simulink model "elaborated_design"  (Simulink 7.0)
settings: Solver=ode45  SolverMode=SingleTasking  StartTime=0.0  StopTime=24/3000  RelTol=1e-6
PreLoadFcn:
  | load one_stage.mat
  | load multi_stage.mat
  | generate_fir_lut
undefined symbols (not defined in the file or in its folder): hm, lut_matrix
libraries: simulink x9, dspmlti4 x4, simulink_extras x2, dspsigops x1
(part 1 of 2)
settings Model: Creator=abehbood  LastModifiedBy=abehbood  BufferReuse=off
settings SolverCC: ConsecutiveZCsStepRelTol=128*eps  ZeroCrossControl=DisableAll
settings DataIOCC: LimitDataPoints=off  SaveFormat=StructureWithTime
settings OptimizationCC: OptimizeBlockIOStorage=off  BufferReuse=off  ExpressionFolding=off  LocalBlockOutputs=off
settings DebuggingCC: SaveWithParameterizedLinksMsg=none  SignalResolutionControl=TryResolveAllWithWarning
settings GRTTargetCC: TargetFcnLib=ansi_tfl_tmw.mat

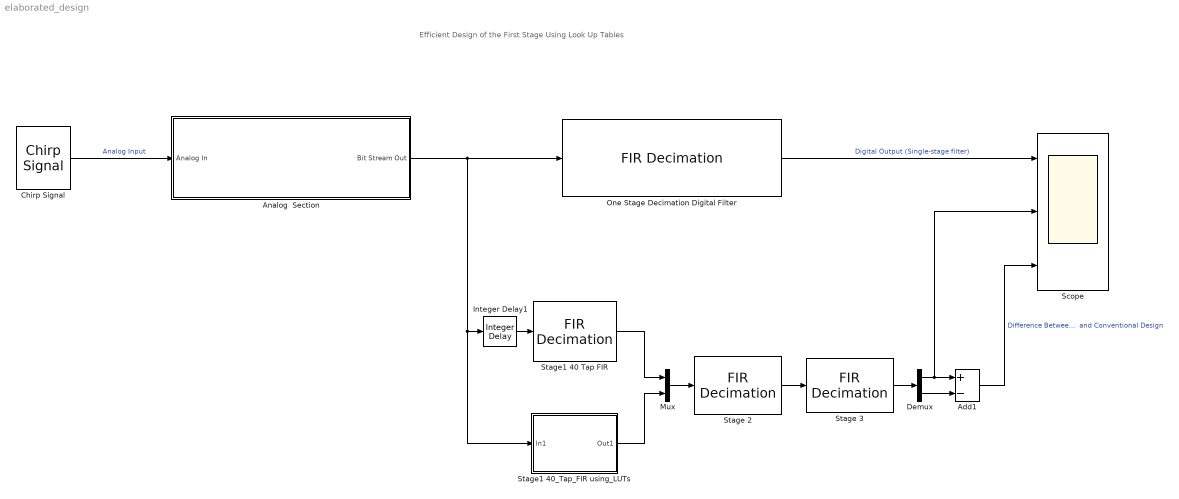
== system elaborated_design ==
  note: Efficient Design of the First Stage
      | Using Look Up Tables
  Add1 : Sum  Inputs=+-  OutDataType=sfix(16)  OutScaling=2^-10
  Analog  Section : Subsystem
  Chirp Signal : simulink/Sources/Chirp Signal  SystemSampleTime=-1  f1=.1  T=6/3000  f2=1000
  Demux : Demux  Outputs=2
  Integer Delay1 : simulink/Discrete/Integer Delay  vinit=0  samptime=-1  NumDelays=1
  Mux : Mux  Inputs=2
  One Stage Decimation Digital Filter : dspmlti4/FIR Decimation  Tag=BlockMethodSubSystem  RequirementInfo={'other' 'AD1877.pdf' '#4' 'true' 'ADI AD1877 Data Sheet' '' } %GIDa_09ac136c_1eca_41b1_bc0b_62c1f7d0b7d0  DialogController=dspdialog.FIRDecimation  DialogControllerArgs=DataTag0  h=[1.55406407911568e-005 -4.02976869344532e-006 -3.62744882919974e-006 -3.32415900794419e-006 -3.10004007346292e-006 -2.94488775900927e-006 -2.84407867825443e-006 -2.79175810569639e-006 -2.77680534274625e-006 -2.79636876946116e-006 -2.84159739559419e-006 -2.91172216432913e-006 -2.99938731666961e-006 -3.10526988821609e-006 -3.22293122491583e-006 -3.35411175577608e-006 -3.49288760841827e-006 -3.64182441067023e-006 -3.79519422790614e-006 -3.95625120366779e-006 -4.11924776887857e-006 -4.28807690784027e-006 -4.45674935295447e-006 -4.62985561457222e-006 -4.800897058436e-006 -4.9753188968358e-006 -5.14579209170125e-006 -5.31896147362731e-006 -5.48613787011061e-006 -5.65584148286576e-006 -5.81687994870294e-006 -5.98156442936665e-006 -6.1319779994032e-006 -6.29670705116336e-006 -6.41916030653874e-006 -6.5873274394144e-006 -6.7177176233061e-006 -6.82652503989139e-006 -6.95495460798152e-006 -7.07534295461106e-006 -7.1850354195168e-006 -7.27502374181979e-006 -7.35666591949478e-006 -7.42908966098812e-006 -7.49731879243244e-006 -7.55554016300166e-006 -7.60384694343128e-006 -7.63736428406282e-006 -7.65751209128601e-006 -7.66271823557677e-006 -7.65541155261304e-006 -7.63501627507501e-006 -7.60282107295533e-006 -7.55771586095076e-006 -7.49955110139743e-006 -7.42707797821989e-006 -7.33956971085392e-006 -7.23653893398005e-006 -7.11727392514411e-006 -6.98238367840012e-006 -6.83104946879514e-006 -6.66483440906746e-006 -6.48225897487408e-006 -6.28578538645417e-006 -6.07254142810829e-006 -5.84668058135014e-006 -5.60212405026277e-006 -5.34827643472346e-006 -5.07102301413336e-006 -4.78659690402004e-006 -4.48580556034723e-006 -4.16155600384522e-006 -3.83401955134294e-006 -3.48874328670483e-006 -3.12800075717904e-006 -2.75159431264472e-006 -2.36710798789534e-006 -1.97052071697094e-006 -1.56289826517329e-006 -1.1415501968765e-006 -7.10846494538715e-007 -2.70732289220279e-007 1.75793679903884e-007 6.30605543525479e-007 1.09226506478532e-006 1.56189731593155e-006 2.03697170915753e-006 2.51723717113145e-006 3.00015723143587e-006 3.48579071809432e-006 3.9725933377886e-006 4.46080384428176e-006 4.9490441253173e-006 5.43679761975195e-006 5.92239585030302e-006 6.40461366377309e-006 6.88208470617973e-006 7.35331974962638e-006 7.81788083672163e-006 8.27366149467831e-006 8.72161880365281e-006 9.15789014754869e-006 9.58466277051695e-006 9.99868488513386e-006 1.03961241773662e-005 1.07845165019174e-005 1.11507237228684e-005 1.1501595755956e-005 1.18347779752421e-005 1.21491508417921e-005 1.24402661260835e-005 1.27113476734474e-005 1.29603423782727e-005 1.31870907689413e-005 1.33876586413025e-005 1.35630197026232e-005 1.37115784405412e-005 1.38343308497875e-005 1.39285220410779e-005 1.39941223446797e-005 1.40289966823036e-005 1.40342134443906e-005 1.40084936488381e-005 1.39526353305602e-005 1.3864821369379e-005 1.37453066068296e-005 1.35925703287186e-005 1.34073463479953e-005 1.3188789625357e-005 1.29377174450497e-005 1.26533131128865e-005 1.23359924862388e-005 1.19851377636711e-005 1.16010858578809e-005 1.11839953027825e-005 1.07344849783013e-005 1.02524591509204e-005 9.74071213530745e-006 9.19501972815777e-006 8.62303106439748e-006 8.0182133965873e-006 7.38519650181956e-006 6.72464037253548e-006 6.03717286198122e-006 5.32193639834688e-006 4.58308951056204e-006 3.82060966862603e-006 3.03594631004846e-006 2.22877471347222e-006 1.40249577164911e-006 5.57771396078279e-007 -3.03081212010611e-007 -1.18011136255105e-006 -2.0703284116168e-006 -2.97257001796215e-006 -3.8836096780257e-006 -4.80290798314314e-006 -5.72785477296596e-006 -6.65770229898759e-006 -7.58923677050474e-006 -8.52121235074221e-006 -9.45049303838782e-006 -1.03761550722017e-005 -1.12952557815384e-005 -1.22066400703126e-005 -1.31069929510391e-005 -1.39948646063552e-005 -1.48669844016962e-005 -1.5722291797911e-005 -1.6557361960285e-005 -1.73721743499725e-005 -1.81614198379814e-005 -1.89271227804299e-005 -1.96621709077627e-005 -2.03681220570147e-005 -2.10414746689456e-005 -2.16795973059757e-005 ...(+43466 chars)]  D=64  filtStruct=Direct form  framing=Maintain input frame size  outputBufInitCond=0  roundingMode=Floor  overflowMode=off  FilterSource=Filter object  FilterObject=h
  Scope : Scope  NumInputPorts=3
      settings: TimeRange=0.008  YMin=-2~-2~-0.2  YMax=2~2~0.2
  Stage 2 : dspmlti4/FIR Decimation  Tag=BlockMethodSubSystem  DialogController=dspdialog.FIRDecimation  DialogControllerArgs=DataTag1  h=[0.006011962890625 -0.0025787353515625 -0.0494384765625 0.0092315673828125 0.293411254882813 0.486648559570313 0.293411254882813 0.0092315673828125 -0.0494384765625 -0.0025787353515625 0.006011962890625]  D=2  filtStruct=Direct form  framing=Maintain input frame size  outputBufInitCond=0  firstCoeffMode=Binary point scaling  firstCoeffWordLength=16  firstCoeffFracLength=16  outputMode=Binary point scaling  outputWordLength=16  outputFracLength=15  accumMode=Binary point scaling  accumWordLength=33  accumFracLength=31  prodOutputMode=Binary point scaling  prodOutputWordLength=31  prodOutputFracLength=31  roundingMode=Nearest  overflowMode=off  FilterSource=Filter object  FilterObject=hm.stage(2)
  Stage 3 : dspmlti4/FIR Decimation  Tag=BlockMethodSubSystem  DialogController=dspdialog.FIRDecimation  DialogControllerArgs=DataTag2  h=[-2.288818359375e-005 -7.62939453125e-006 1.52587890625e-005 4.57763671875e-005 8.392333984375e-005 8.392333984375e-005 3.814697265625e-005 -5.340576171875e-005 -0.0001373291015625 -0.0001678466796875 -9.918212890625e-005 5.340576171875e-005 0.0002288818359375 0.00031280517578125 0.00022125244140625 -3.0517578125e-005 -0.000335693359375 -0.000518798828125 -0.00043487548828125 -6.103515625e-005 0.00045013427734375 0.0008087158203125 0.00077056884765625 0.00025177001953125 -0.00054168701171875 -0.0011749267578125 -0.001251220703125 -0.000579833984375 0.00057220458984375 0.001617431640625 0.0019073486328125 0.0011138916015625 -0.00048828125 -0.002105712890625 -0.00276947021484375 -0.00191497802734375 0.0002288818359375 0.0026092529296875 0.0038604736328125 0.0030517578125 0.00031280517578125 -0.0030670166015625 -0.00519561767578125 -0.0046234130859375 -0.0012359619140625 0.00341033935546875 0.00679779052734375 0.006744384765625 0.00272369384765625 -0.00353240966796875 -0.008697509765625 -0.00959014892578125 -0.00499725341796875 0.00327301025390625 0.0109710693359375 0.0134963989257813 0.0084991455078125 -0.00238037109375 -0.0137939453125 -0.0191268920898438 -0.01409912109375 0.0003662109375 0.0176849365234375 0.028228759765625 0.0241317749023438 0.0041046142578125 -0.0243759155273438 -0.0468978881835938 -0.0477294921875 -0.0169906616210938 0.0438156127929688 0.120735168457031 0.191574096679688 0.233955383300781 0.233955383300781 0.191574096679688 0.120735168457031 0.0438156127929688 -0.0169906616210938 -0.0477294921875 -0.0468978881835938 -0.0243759155273438 0.0041046142578125 0.0241317749023438 0.028228759765625 0.0176849365234375 0.0003662109375 -0.01409912109375 -0.0191268920898438 -0.0137939453125 -0.00238037109375 0.0084991455078125 0.0134963989257813 0.0109710693359375 0.00327301025390625 -0.00499725341796875 -0.00959014892578125 -0.008697509765625 -0.00353240966796875 0.00272369384765625 0.006744384765625 0.00679779052734375 0.00341033935546875 -0.0012359619140625 -0.0046234130859375 -0.00519561767578125 -0.0030670166015625 0.00031280517578125 0.0030517578125 0.0038604736328125 0.0026092529296875 0.0002288818359375 -0.00191497802734375 -0.00276947021484375 -0.002105712890625 -0.00048828125 0.0011138916015625 0.0019073486328125 0.001617431640625 0.00057220458984375 -0.000579833984375 -0.001251220703125 -0.0011749267578125 -0.00054168701171875 0.00025177001953125 0.00077056884765625 0.0008087158203125 0.00045013427734375 -6.103515625e-005 -0.00043487548828125 -0.000518798828125 -0.000335693359375 -3.0517578125e-005 0.00022125244140625 0.00031280517578125 0.0002288818359375 5.340576171875e-005 -9.918212890625e-005 -0.0001678466796875 -0.0001373291015625 -5.340576171875e-005 3.814697265625e-005 8.392333984375e-005 8.392333984375e-005 4.57763671875e-005 1.52587890625e-005 -7.62939453125e-006 -2.288818359375e-005]  D=4  filtStruct=Direct form  framing=Maintain input frame size  outputBufInitCond=0  firstCoeffMode=Binary point scaling  firstCoeffWordLength=16  firstCoeffFracLength=17  outputMode=Binary point scaling  outputWordLength=16  outputFracLength=15  accumMode=Binary point scaling  accumWordLength=34  accumFracLength=32  prodOutputMode=Binary point scaling  prodOutputWordLength=31  prodOutputFracLength=32  roundingMode=Nearest  overflowMode=off  FilterSource=Filter object  FilterObject=hm.stage(3)
  Stage1 40 Tap FIR : dspmlti4/FIR Decimation  Tag=BlockMethodSubSystem  DialogController=dspdialog.FIRDecimation  DialogControllerArgs=DataTag3  h=[-9.5367431640625e-005 -0.00032806396484375 -0.00081634521484375 -0.00164794921875 -0.00287246704101563 -0.004425048828125 -0.00608062744140625 -0.007415771484375 -0.0078125 -0.0065155029296875 -0.00275421142578125 0.00410842895507813 0.0143890380859375 0.0279426574707031 0.0440788269042969 0.0615692138671875 0.0787696838378906 0.0938453674316406 0.105056762695313 0.111034393310547 0.111034393310547 0.105056762695313 0.0938453674316406 0.0787696838378906 0.0615692138671875 0.0440788269042969 0.0279426574707031 0.0143890380859375 0.00410842895507813 -0.00275421142578125 -0.0065155029296875 -0.0078125 -0.007415771484375 -0.00608062744140625 -0.004425048828125 -0.00287246704101563 -0.00164794921875 -0.00081634521484375 -0.00032806396484375 -9.5367431640625e-005]  D=8  filtStruct=Direct form  framing=Maintain input frame size  outputBufInitCond=0  firstCoeffMode=Binary point scaling  firstCoeffWordLength=16  firstCoeffFracLength=18  outputMode=Binary point scaling  outputWordLength=16  outputFracLength=15  accumMode=Binary point scaling  accumWordLength=20  accumFracLength=18  prodOutputMode=Binary point scaling  prodOutputWordLength=16  prodOutputFracLength=18  roundingMode=Nearest  overflowMode=off  FilterSource=Filter object  FilterObject=hm.stage(1)
  Stage1 40_Tap_FIR using_LUTs : Subsystem
  wires:
  One Stage Decimation Digital Filter/1 -> Scope/1  "Digital Output (Single-stage filter)"
  Analog  Section/1(Bit Stream Out) -> One Stage Decimation Digital Filter/1, Integer Delay1/1, Stage1 40_Tap_FIR using_LUTs/1(In1)
  Chirp Signal/1 -> Analog  Section/1(Analog In)  "Analog Input"
  Stage1 40_Tap_FIR using_LUTs/1(Out1) -> Mux/2
  Stage1 40 Tap FIR/1 -> Mux/1
  Stage 2/1 -> Stage 3/1
  Integer Delay1/1 -> Stage1 40 Tap FIR/1
  Stage 3/1 -> Demux/1
  Demux/1 -> Add1/1, Scope/2
  Demux/2 -> Add1/2
  Mux/1 -> Stage 2/1
  Add1/1 -> Scope/3  "Difference Between LUT Design  and Conventional Design"
